simulink model "LqtSimulink2018a"  (R2018a)
settings: Solver=VariableStepAuto  StartTime=0.0  StopTime=10  RelTol=1e-3
values from neighbouring files (symbols this model uses):
  A_d = sys_d.A    [progetto.m]
  B_d = sys_d.B    [progetto.m]
  C = eye(4)    [progetto.m]
  D = zeros(4,1)    [progetto.m]
  t_sample = 0.01    [progetto.m]
  x0 = [2 6.25 -pi/2 0]'    [progetto.m]
settings Model: Creator=carda  LastModifiedBy=stela
settings DataIOCC: ReturnWorkspaceOutputs=on
settings SFSimCC: SimUseLocalCustomCode=on
settings RTWCC: RTWUseLocalCustomCode=on

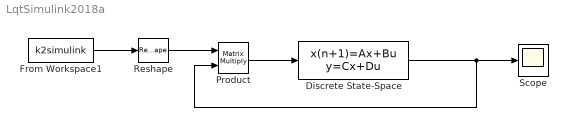
== system LqtSimulink2018a ==
  Discrete State-Space : DiscreteStateSpace  A=A_d  B=B_d  C=C  D=D  InitialCondition=x0  SampleTime=t_sample
  From Workspace1 : FromWorkspace  VariableName=k2simulink  SampleTime=1
  Product : Product  Multiplication=Matrix(*)
  Reshape : Reshape  OutputDimensionality=Customize  OutputDimensions=[1,4]
  Scope : Scope
  wires:
  Discrete State-Space/1 -> Product/2, Scope/1
  Reshape/1 -> Product/1
  From Workspace1/1 -> Reshape/1
  Product/1 -> Discrete State-Space/1
